simulink model "FixedWing_Dynamic_Model_SIL_simulink"  (R2023a)
settings: Solver=ode4  StartTime=0.0  StopTime=timestop  FixedStep=0.004  RelTol=1e-3
model workspace (MAT data in the model file):
  sample_time = 0.004
values from neighbouring files (symbols this model uses):
  env = struct    [InitEnvironment.m]    (also in resultados_autotuning_H200.mat = )
  F_lat = 1    [autotuning.m]    (also in resultados_autotuning_H200.mat)
  F_lon = 1    [autotuning.m]    (also in resultados_autotuning_H200.mat)
  frecuency = 0.012    [PX4_var_controllers.m]    (also in resultados_autotuning_H200.mat)
  g = 9.81    [PX4_var_controllers.m]    (also in resultados_autotuning_H200.mat)
  LC =     [resultados_autotuning_H200.mat]
  mission = [wp]    [PX4_var_controllers.m]    (also in resultados_autotuning_H200.mat = )
  nav = 0    [autotuning.m]    (also in resultados_autotuning_H200.mat)
  nwap = 9    [PX4_var_controllers.m]    (also in resultados_autotuning_H200.mat)
  pitch_D = p(8)    [Error_Medio_Cuadratico_tot.m]    (also in autotuning.m = gaDat3.xmin(8); resultados_autotuning_H200.mat = 0.0563748318956)
  pitch_ff = p(10)    [Error_Medio_Cuadratico_tot.m]    (also in autotuning.m = gaDat3.xmin(10); resultados_autotuning_H200.mat = 0.191071934851)
  pitch_I = p(7)    [Error_Medio_Cuadratico_tot.m]    (also in autotuning.m = gaDat3.xmin(7); resultados_autotuning_H200.mat = 5.51002123548)
  pitch_P = p(6)    [Error_Medio_Cuadratico_tot.m]    (also in autotuning.m = gaDat3.xmin(6); resultados_autotuning_H200.mat = 0.842081867818)
  poswp = [poswp1;poswp2;poswp3;poswp4;poswp5;poswp6;poswp7;poswp8;poswp9]    [PX4_var_controllers.m]    (also in resultados_autotuning_H200.mat = [0 203.689232032 39.9384744604 259.790159417 479.641844374 3)
  ref_height = 171    [resultados_autotuning_H200.mat]
  ref_lat = 39.4973880749    [resultados_autotuning_H200.mat]
  ref_lon = -0.626812248872    [resultados_autotuning_H200.mat]
  roll_D = p(3)    [Error_Medio_Cuadratico_lat.m]    (also in Error_Medio_Cuadratico_tot.m; autotuning.m = gaDat3.xmin(3); resultados_autotuning_H200.mat = 0.0337053005157)
  roll_ff = p(5)    [Error_Medio_Cuadratico_lat.m]    (also in Error_Medio_Cuadratico_tot.m; autotuning.m = gaDat3.xmin(5); resultados_autotuning_H200.mat = 0.350805641616)
  roll_I = p(2)    [Error_Medio_Cuadratico_lat.m]    (also in Error_Medio_Cuadratico_tot.m; autotuning.m = gaDat3.xmin(2); resultados_autotuning_H200.mat = 5.74910821603)
  roll_P = p(1)    [Error_Medio_Cuadratico_lat.m]    (also in Error_Medio_Cuadratico_tot.m; autotuning.m = gaDat3.xmin(1); resultados_autotuning_H200.mat = 0.613573974385)
  tc_pitch = p(9)    [Error_Medio_Cuadratico_tot.m]    (also in autotuning.m = gaDat3.xmin(9); resultados_autotuning_H200.mat = 0.651709962584)
  tc_roll = p(4)    [Error_Medio_Cuadratico_lat.m]    (also in Error_Medio_Cuadratico_tot.m; autotuning.m = gaDat3.xmin(4); resultados_autotuning_H200.mat = 0.630975334126)
  TEBCL =     [resultados_autotuning_H200.mat]
  TECL =     [resultados_autotuning_H200.mat]
  TECS =     [resultados_autotuning_H200.mat]
  throttle_sp = 0.6    [autotuning.m]    (also in resultados_autotuning_H200.mat)
  uavData = struct    [InitFixedWingParam.m]    (also in resultados_autotuning_H200.mat = )
  V_cruise = [15,15,15,20,25,25,20,15,15]    [PX4_var_controllers.m]    (also in resultados_autotuning_H200.mat = [15 15 15 20 25 25 20 15 15])
  yaw_D = p(8)    [Error_Medio_Cuadratico_lat.m]    (also in Error_Medio_Cuadratico_tot.m = p(13); autotuning.m = gaDat3.xmin(13); resultados_autotuning_H200.mat = 0.366142516918)
  yaw_ff = p(9)    [Error_Medio_Cuadratico_lat.m]    (also in Error_Medio_Cuadratico_tot.m = p(14); autotuning.m = gaDat3.xmin(14); resultados_autotuning_H200.mat = 1.32395168)
  yaw_I = p(7)    [Error_Medio_Cuadratico_lat.m]    (also in Error_Medio_Cuadratico_tot.m = p(12); autotuning.m = gaDat3.xmin(12); resultados_autotuning_H200.mat = 9.97252106698)
  yaw_P = p(6)    [Error_Medio_Cuadratico_lat.m]    (also in Error_Medio_Cuadratico_tot.m = p(11); autotuning.m = gaDat3.xmin(11); resultados_autotuning_H200.mat = 9.79447138521)
undefined symbols (not defined in the file or in its folder): DiscIntNeverNeededParam, Earth, WGS84
libraries: aerolibactuator x5, aerolibasang x4, slpidlib x3, uavalgslib x2, aerolibatmos2 x2, shared6dof x1, aerolibtransform2 x1, simulink_extras x1
(part 3 of 3)

== system FixedWing_Dynamic_Model_SIL_simulink/Dynamics/H200 Fixed-wing UAV Dynamics/Force and Moment Calculation/Motor Model/Engine Model/Thurst Model/N [Hz] model ==
  deltaP : Inport
  " " : Gain  Gain=uavData.engine.propellerModel.RPMModel.pn1
  Saturation : Saturate  UpperLimit=1  LowerLimit=0
  n : Outport
  wires:
  " "/1 -> n/1
  deltaP/1 -> Saturation/1
  Saturation/1 -> " "/1

== system FixedWing_Dynamic_Model_SIL_simulink/Dynamics/H200 Fixed-wing UAV Dynamics/Force and Moment Calculation/Motor Model/Engine Model/Thurst Model/Thrust Force ==
  n : Inport
  CT : Inport  Port=2
  rho : Inport  Port=3
  Constant : Constant  Value=uavData.engine.bladeDiameter
  Constant1 : Constant  Value=4
  Power : Math  Operator=pow
  Product : Product  Inputs=4
  Square : Math  Operator=square
  T : Outport
  wires:
  Constant/1 -> Power/1
  n/1 -> Square/1
  Square/1 -> Product/1
  CT/1 -> Product/2
  rho/1 -> Product/3
  Product/1 -> T/1
  Power/1 -> Product/4
  Constant1/1 -> Power/2

== system FixedWing_Dynamic_Model_SIL_simulink/Dynamics/H200 Fixed-wing UAV Dynamics/Force and Moment Calculation/Aerodynamic Forces and Moments/Compute Body Frame Forces and Moments/Rotate FM to body frame/Rotate Forces/RB2W ==
  aoa beta : Inport
  11 : Fcn  Expr=u[3]*u[4]
  12 : Fcn  Expr=u[2]
  13 : Fcn  Expr=u[1]*u[4]
  21 : Fcn  Expr=-u[3]*u[2]
  22 : Fcn  Expr=u[4]
  23 : Fcn  Expr=-u[1]*u[2]
  31 : Fcn  Expr=-u[1]
  32 : Fcn  Expr=0
  33 : Fcn  Expr=u[3]
  Mux : Mux  Inputs=2
  Mux3 : Mux  Inputs=9
  Reshape 9x1->3x3 : Reshape  OutputDimensionality=Customize  OutputDimensions=[3,3]
  sincos : Trigonometry  Operator=sincos
  Rw2b : Outport  VectorParamsAs1DForOutWhenUnconnected=off
  wires:
  Mux/1 -> 11/1, 21/1, 31/1, 12/1, 22/1, 32/1, 13/1, 23/1, 33/1
  aoa beta/1 -> sincos/1
  sincos/2 -> Mux/2
  sincos/1 -> Mux/1
  33/1 -> Mux3/9
  23/1 -> Mux3/8
  13/1 -> Mux3/7
  32/1 -> Mux3/6
  22/1 -> Mux3/5
  12/1 -> Mux3/4
  31/1 -> Mux3/3
  21/1 -> Mux3/2
  11/1 -> Mux3/1
  Reshape 9x1->3x3/1 -> Rw2b/1
  Mux3/1 -> Reshape 9x1->3x3/1

== system FixedWing_Dynamic_Model_SIL_simulink/Dynamics/H200 Fixed-wing UAV Dynamics/Force and Moment Calculation/Aerodynamic Forces and Moments/Compute Body Frame Forces and Moments/Rotate FM to body frame/Rotate Moments/RB2W ==
  aoa beta : Inport
  11 : Fcn  Expr=u[3]*u[4]
  12 : Fcn  Expr=u[2]
  13 : Fcn  Expr=u[1]*u[4]
  21 : Fcn  Expr=-u[3]*u[2]
  22 : Fcn  Expr=u[4]
  23 : Fcn  Expr=-u[1]*u[2]
  31 : Fcn  Expr=-u[1]
  32 : Fcn  Expr=0
  33 : Fcn  Expr=u[3]
  Mux : Mux  Inputs=2
  Mux3 : Mux  Inputs=9
  Reshape 9x1->3x3 : Reshape  OutputDimensionality=Customize  OutputDimensions=[3,3]
  sincos : Trigonometry  Operator=sincos
  Rw2b : Outport  VectorParamsAs1DForOutWhenUnconnected=off
  wires:
  Mux/1 -> 11/1, 21/1, 31/1, 12/1, 22/1, 32/1, 13/1, 23/1, 33/1
  aoa beta/1 -> sincos/1
  sincos/2 -> Mux/2
  sincos/1 -> Mux/1
  33/1 -> Mux3/9
  23/1 -> Mux3/8
  13/1 -> Mux3/7
  32/1 -> Mux3/6
  22/1 -> Mux3/5
  12/1 -> Mux3/4
  31/1 -> Mux3/3
  21/1 -> Mux3/2
  11/1 -> Mux3/1
  Reshape 9x1->3x3/1 -> Rw2b/1
  Mux3/1 -> Reshape 9x1->3x3/1

== system FixedWing_Dynamic_Model_SIL_simulink/Dynamics/H200 Fixed-wing UAV Dynamics/Force and Moment Calculation/Aerodynamic Forces and Moments/Compute Body Frame Forces and Moments/Wind frame F& M/Lateral Channel/CY ==
  beta : Inport
  p,q,r : Inport  Port=2
  Airspeed : Inport  Port=3
  deltaR : Inport  Port=4
  deltaA : Inport  Port=5
  CYDr : Constant  Value=uavData.aero.CYdeltaR
      settings: AttributesFormatString=%<Value>
  CYDr1 : Constant  Value=uavData.aero.CYdeltaA
      settings: AttributesFormatString=%<Value>
  CYb : Constant  Value=uavData.aero.CYbeta
      settings: AttributesFormatString=%<Value>
  Product : Product  SaturateOnIntegerOverflow=on  OutDataTypeStr=Inherit: Same as first input
  Product1 : Product  SaturateOnIntegerOverflow=on  OutDataTypeStr=Inherit: Same as first input
  Product2 : Product  SaturateOnIntegerOverflow=on  OutDataTypeStr=Inherit: Same as first input
  Sum2 : Sum  Inputs=+++++  SaturateOnIntegerOverflow=on
  roll / yaw rate factors : Subsystem
  CY : Outport  VectorParamsAs1DForOutWhenUnconnected=off
  wires:
  deltaR/1 -> Product1/2
  CYDr/1 -> Product1/1
  Product/1 -> Sum2/1
  Sum2/1 -> CY/1
  beta/1 -> Product/2
  CYb/1 -> Product/1
  CYDr1/1 -> Product2/1
  deltaA/1 -> Product2/2
  Product2/1 -> Sum2/5
  Product1/1 -> Sum2/4
  roll / yaw rate factors/1(CYp) -> Sum2/2
  roll / yaw rate factors/2(CYr) -> Sum2/3
  p,q,r/1 -> roll / yaw rate factors/1(p,q,r)
  Airspeed/1 -> roll / yaw rate factors/2(Airspeed)

== system FixedWing_Dynamic_Model_SIL_simulink/Dynamics/H200 Fixed-wing UAV Dynamics/Force and Moment Calculation/Aerodynamic Forces and Moments/Compute Body Frame Forces and Moments/Wind frame F& M/Lateral Channel/Cl ==
  beta : Inport
  p,q,r : Inport  Port=2
  Airspeed : Inport  Port=3
  deltaR : Inport  Port=4
  deltaA : Inport  Port=5
  CYDr : Constant  Value=uavData.aero.CldeltaR
      settings: AttributesFormatString=%<Value>
  CYDr1 : Constant  Value=uavData.aero.CldeltaA
      settings: AttributesFormatString=%<Value>
  Clb : Constant  Value=uavData.aero.Clbeta
      settings: AttributesFormatString=%<Value>
  Product2 : Product  SaturateOnIntegerOverflow=on  OutDataTypeStr=Inherit: Same as first input
  Product3 : Product  SaturateOnIntegerOverflow=on  OutDataTypeStr=Inherit: Same as first input
  Product4 : Product  SaturateOnIntegerOverflow=on  OutDataTypeStr=Inherit: Same as first input
  Sum : Sum  Inputs=+++++  SaturateOnIntegerOverflow=on
  roll factors : Subsystem
  Cl : Outport  VectorParamsAs1DForOutWhenUnconnected=off
  wires:
  Airspeed/1 -> roll factors/2(Airspeed)
  p,q,r/1 -> roll factors/1(p,q,r)
  Product4/1 -> Sum/1  "Clb"
  Sum/1 -> Cl/1
  beta/1 -> Product4/2
  Clb/1 -> Product4/1
  CYDr1/1 -> Product3/1
  deltaR/1 -> Product2/2
  deltaA/1 -> Product3/2
  Product2/1 -> Sum/4
  CYDr/1 -> Product2/1
  Product3/1 -> Sum/5
  roll factors/1(Clp) -> Sum/2
  roll factors/2(Clr) -> Sum/3

== system FixedWing_Dynamic_Model_SIL_simulink/Dynamics/H200 Fixed-wing UAV Dynamics/Force and Moment Calculation/Aerodynamic Forces and Moments/Compute Body Frame Forces and Moments/Wind frame F& M/Lateral Channel/Cn ==
  beta : Inport
  p,q,r : Inport  Port=2
  Airspeed : Inport  Port=3
  deltaR : Inport  Port=4
  deltaA : Inport  Port=5
  CnDa : Constant  Value=uavData.aero.CndeltaA
      settings: AttributesFormatString=%<Value>
  CnDr : Constant  Value=uavData.aero.CndeltaR
      settings: AttributesFormatString=%<Value>
  Cnb : Constant  Value=uavData.aero.Cnbeta
      settings: AttributesFormatString=%<Value>
  Product2 : Product  SaturateOnIntegerOverflow=on  OutDataTypeStr=Inherit: Same as first input
  Product3 : Product  SaturateOnIntegerOverflow=on  OutDataTypeStr=Inherit: Same as first input
  Product4 : Product  SaturateOnIntegerOverflow=on  OutDataTypeStr=Inherit: Same as first input
  Sum : Sum  Inputs=+++++  SaturateOnIntegerOverflow=on
  roll / yaw rate factors : Subsystem
  Cn : Outport  VectorParamsAs1DForOutWhenUnconnected=off
  wires:
  Airspeed/1 -> roll / yaw rate factors/2(Airspeed)
  p,q,r/1 -> roll / yaw rate factors/1(p,q,r)
  Cnb/1 -> Product4/1
  beta/1 -> Product4/2
  Sum/1 -> Cn/1
  Product4/1 -> Sum/1
  roll / yaw rate factors/1(Cnp) -> Sum/2
  roll / yaw rate factors/2(Cnr) -> Sum/3
  deltaR/1 -> Product2/2
  CnDr/1 -> Product2/1
  CnDa/1 -> Product3/1
  deltaA/1 -> Product3/2
  Product2/1 -> Sum/4
  Product3/1 -> Sum/5

== system FixedWing_Dynamic_Model_SIL_simulink/Dynamics/H200 Fixed-wing UAV Dynamics/Force and Moment Calculation/Aerodynamic Forces and Moments/Compute Body Frame Forces and Moments/Wind frame F& M/Longitudinal Channel/CD ==
  CL : Inport
  Apolar : Constant  Value=uavData.aero.A1
      settings: AttributesFormatString=%<Value>
  Apolar (A2) : Constant  Value=uavData.aero.Apolar
      settings: AttributesFormatString=%<Value>
  CD0 : Constant  Value=uavData.aero.CD0
      settings: AttributesFormatString=%<Value>
  Math Function : Math  Operator=square  SignedPower=on
  Product : Product  SaturateOnIntegerOverflow=on  OutDataTypeStr=Inherit: Same as first input
  Product1 : Product  SaturateOnIntegerOverflow=on  OutDataTypeStr=Inherit: Same as first input
  Sum1 : Sum  Inputs=+++  SaturateOnIntegerOverflow=on
  CD : Outport  VectorParamsAs1DForOutWhenUnconnected=off
  wires:
  Sum1/1 -> CD/1
  Apolar (A2)/1 -> Product/1
  Math Function/1 -> Product/2
  Product1/1 -> Sum1/3
  Product/1 -> Sum1/2
  CL/1 -> Math Function/1, Product1/1
  CD0/1 -> Sum1/1
  Apolar/1 -> Product1/2

== system FixedWing_Dynamic_Model_SIL_simulink/Dynamics/H200 Fixed-wing UAV Dynamics/Force and Moment Calculation/Aerodynamic Forces and Moments/Compute Body Frame Forces and Moments/Wind frame F& M/Longitudinal Channel/CL ==
  alpha : Inport
  alpha_dot : Inport  Port=2
  p,q,r : Inport  Port=3
  Airspeed : Inport  Port=4
  deltaE : Inport  Port=5
  deltaF : Inport  Port=6
  AoA rate / pitch rate factors : Subsystem
  CL0 : Constant  Value=uavData.aero.CL0
      settings: AttributesFormatString=%<Value>
  CLDe : Constant  Value=uavData.aero.CLdeltaE
      settings: AttributesFormatString=%<Value>
  CLa : Constant  Value=uavData.aero.CLalpha
      settings: AttributesFormatString=%<Value>
  CmDe1 : Constant  Value=uavData.aero.CLdeltaF
      settings: AttributesFormatString=%<Value>
  Product1 : Product  SaturateOnIntegerOverflow=on  OutDataTypeStr=Inherit: Same as first input
  Product3 : Product  SaturateOnIntegerOverflow=on  OutDataTypeStr=Inherit: Same as first input
  Product4 : Product  SaturateOnIntegerOverflow=on  OutDataTypeStr=Inherit: Same as first input
  Sum : Sum  Inputs=++++++  SaturateOnIntegerOverflow=on
  CL : Outport  VectorParamsAs1DForOutWhenUnconnected=off
  wires:
  CL0/1 -> Sum/1  "CL0"
  deltaF/1 -> Product3/2
  Sum/1 -> CL/1
  deltaE/1 -> Product1/2
  CLDe/1 -> Product1/1
  alpha/1 -> Product4/2
  CLa/1 -> Product4/1
  Product4/1 -> Sum/2  "CLalpha"
  alpha_dot/1 -> AoA rate / pitch rate factors/1(alpha_dot)
  Airspeed/1 -> AoA rate / pitch rate factors/3(Airspeed)
  p,q,r/1 -> AoA rate / pitch rate factors/2(p,q,r)
  AoA rate / pitch rate factors/1(CLalpha_dot) -> Sum/3  "CLapha_dot"
  AoA rate / pitch rate factors/2(CLq) -> Sum/4  "CLq"
  Product1/1 -> Sum/5  "CLdeltaE"
  CmDe1/1 -> Product3/1
  Product3/1 -> Sum/6  "CLdeltaF"

== system FixedWing_Dynamic_Model_SIL_simulink/Dynamics/H200 Fixed-wing UAV Dynamics/Force and Moment Calculation/Aerodynamic Forces and Moments/Compute Body Frame Forces and Moments/Wind frame F& M/Longitudinal Channel/Cm ==
  alpha : Inport
  alpha_dot : Inport  Port=2
  p,q,r : Inport  Port=3
  Airpseed : Inport  Port=4
  deltaE : Inport  Port=5
  deltaF : Inport  Port=6
  AoA rate / pitch rate factors : Subsystem
  Cm0 : Constant  Value=uavData.aero.Cm0
      settings: AttributesFormatString=%<Value>
  CmDe : Constant  Value=uavData.aero.CmdeltaE
      settings: AttributesFormatString=%<Value>
  CmDf : Constant  Value=uavData.aero.CmdeltaF
      settings: AttributesFormatString=%<Value>
  Cma : Constant  Value=uavData.aero.Cmalpha
      settings: AttributesFormatString=%<Value>
  Product1 : Product  Inputs=***/  SaturateOnIntegerOverflow=on  OutDataTypeStr=Inherit: Same as first input
  Product2 : Product  SaturateOnIntegerOverflow=on  OutDataTypeStr=Inherit: Same as first input
  Product4 : Product  SaturateOnIntegerOverflow=on  OutDataTypeStr=Inherit: Same as first input
  Sum : Sum  Inputs=++++++  SaturateOnIntegerOverflow=on
  chord : Constant  Value=uavData.geometry.cw
      settings: AttributesFormatString=%<Value>
  elarm : Constant  Value=uavData.geometry.LElev
      settings: AttributesFormatString=%<Value>
  Cm : Outport  VectorParamsAs1DForOutWhenUnconnected=off
  wires:
  chord/1 -> Product1/4
  elarm/1 -> Product1/3
  Product4/1 -> Sum/2  "cma"
  Sum/1 -> Cm/1  "total"
  deltaE/1 -> Product1/2
  CmDe/1 -> Product1/1
  alpha/1 -> Product4/2
  Cma/1 -> Product4/1
  deltaF/1 -> Product2/2
  CmDf/1 -> Product2/1
  Cm0/1 -> Sum/1  "cm0"
  alpha_dot/1 -> AoA rate / pitch rate factors/1(alpha_dot)
  p,q,r/1 -> AoA rate / pitch rate factors/2(p,q,r)
  Airpseed/1 -> AoA rate / pitch rate factors/3(Airspeed)
  AoA rate / pitch rate factors/1(Cmalpha_dot) -> Sum/3  "Cmalpha_dot"
  AoA rate / pitch rate factors/2(Cmq) -> Sum/4  "Cmq"
  Product1/1 -> Sum/5  "cmde"
  Product2/1 -> Sum/6  "cmdf"

== system FixedWing_Dynamic_Model_SIL_simulink/Dynamics/H200 Fixed-wing UAV Dynamics/Force and Moment Calculation/Aerodynamic Forces and Moments/Compute Body Frame Forces and Moments/Wind frame F& M/Lateral Channel/CY/roll // yaw rate factors ==
  p,q,r : Inport
  Airspeed : Inport  Port=2
  Constant : Constant  Value=uavData.aero.CYp
      settings: AttributesFormatString=%<Value>
  Constant1 : Constant  Value=uavData.aero.CYr
      settings: AttributesFormatString=%<Value>
  Get p : Selector  IndexMode=Zero-based  InputPortWidth=3  IndexOptions=Index vector (dialog)  Indices=0  OutputSizes=[(-2)]
  Get r : Selector  IndexMode=Zero-based  InputPortWidth=3  IndexOptions=Index vector (dialog)  Indices=2  OutputSizes=[(-2)]
  Product : Product  SaturateOnIntegerOverflow=on  OutDataTypeStr=Inherit: Same as first input
  Product1 : Product  SaturateOnIntegerOverflow=on  OutDataTypeStr=Inherit: Same as first input
  roll rate fact : Subsystem
  yaw rate fact : Subsystem
  CYp : Outport  VectorParamsAs1DForOutWhenUnconnected=off
  CYr : Outport  Port=2  VectorParamsAs1DForOutWhenUnconnected=off
  wires:
  Airspeed/1 -> roll rate fact/2(Airspeed), yaw rate fact/2(Airspeed)
  Get r/1 -> yaw rate fact/1(r)
  p,q,r/1 -> Get p/1, Get r/1
  Get p/1 -> roll rate fact/1(p)
  roll rate fact/1(Roll Rate Fac) -> Product/2
  Constant/1 -> Product/1
  yaw rate fact/1(Yaw Rate Fac) -> Product1/2
  Constant1/1 -> Product1/1
  Product1/1 -> CYr/1
  Product/1 -> CYp/1

== system FixedWing_Dynamic_Model_SIL_simulink/Dynamics/H200 Fixed-wing UAV Dynamics/Force and Moment Calculation/Aerodynamic Forces and Moments/Compute Body Frame Forces and Moments/Wind frame F& M/Lateral Channel/Cl/roll factors ==
  p,q,r : Inport
  Airspeed : Inport  Port=2
  Constant : Constant  Value=uavData.aero.Clp
      settings: AttributesFormatString=%<Value>
  Constant1 : Constant  Value=uavData.aero.Clr
      settings: AttributesFormatString=%<Value>
  Get p : Selector  IndexMode=Zero-based  InputPortWidth=3  IndexOptions=Index vector (dialog)  Indices=0  OutputSizes=[(-2)]
  Get r : Selector  IndexMode=Zero-based  InputPortWidth=3  IndexOptions=Index vector (dialog)  Indices=2  OutputSizes=[(-2)]
  Product : Product  SaturateOnIntegerOverflow=on  OutDataTypeStr=Inherit: Same as first input
  Product1 : Product  SaturateOnIntegerOverflow=on  OutDataTypeStr=Inherit: Same as first input
  roll rate fact : Subsystem
  yaw rate fact : Subsystem
  Clp : Outport  VectorParamsAs1DForOutWhenUnconnected=off
  Clr : Outport  Port=2  VectorParamsAs1DForOutWhenUnconnected=off
  wires:
  Get r/1 -> yaw rate fact/1(r)
  p,q,r/1 -> Get p/1, Get r/1
  Get p/1 -> roll rate fact/1(p)
  Airspeed/1 -> yaw rate fact/2(Airspeed), roll rate fact/2(Airspeed)
  yaw rate fact/1(Yaw Rate Fac) -> Product1/2
  Constant1/1 -> Product1/1
  roll rate fact/1(Roll Rate Fac) -> Product/2
  Constant/1 -> Product/1
  Product1/1 -> Clr/1
  Product/1 -> Clp/1

== system FixedWing_Dynamic_Model_SIL_simulink/Dynamics/H200 Fixed-wing UAV Dynamics/Force and Moment Calculation/Aerodynamic Forces and Moments/Compute Body Frame Forces and Moments/Wind frame F& M/Lateral Channel/Cn/roll // yaw rate factors ==
  p,q,r : Inport
  Airspeed : Inport  Port=2
  Constant : Constant  Value=uavData.aero.Cnp
      settings: AttributesFormatString=%<Value>
  Constant1 : Constant  Value=uavData.aero.Cnr
      settings: AttributesFormatString=%<Value>
  Get p : Selector  IndexMode=Zero-based  InputPortWidth=3  IndexOptions=Index vector (dialog)  Indices=0  OutputSizes=[(-2)]
  Get r : Selector  IndexMode=Zero-based  InputPortWidth=3  IndexOptions=Index vector (dialog)  Indices=2  OutputSizes=[(-2)]
  Product : Product  SaturateOnIntegerOverflow=on  OutDataTypeStr=Inherit: Same as first input
  Product1 : Product  SaturateOnIntegerOverflow=on  OutDataTypeStr=Inherit: Same as first input
  roll rate fact : Subsystem
  yaw rate fact : Subsystem
  Cnp : Outport  VectorParamsAs1DForOutWhenUnconnected=off
  Cnr : Outport  Port=2  VectorParamsAs1DForOutWhenUnconnected=off
  wires:
  Airspeed/1 -> roll rate fact/2(Airspeed), yaw rate fact/2(Airspeed)
  Get r/1 -> yaw rate fact/1(r)
  p,q,r/1 -> Get p/1, Get r/1
  Get p/1 -> roll rate fact/1(p)
  roll rate fact/1(Roll Rate Fac) -> Product/2
  Constant/1 -> Product/1
  yaw rate fact/1(Yaw Rate Fac) -> Product1/2
  Constant1/1 -> Product1/1
  Product1/1 -> Cnr/1
  Product/1 -> Cnp/1

== system FixedWing_Dynamic_Model_SIL_simulink/Dynamics/H200 Fixed-wing UAV Dynamics/Force and Moment Calculation/Aerodynamic Forces and Moments/Compute Body Frame Forces and Moments/Wind frame F& M/Longitudinal Channel/CL/AoA rate // pitch rate factors ==
  alpha_dot : Inport
  p,q,r : Inport  Port=2
  Airspeed : Inport  Port=3
  AoA rate fact : Subsystem
  Constant : Constant  Value=uavData.aero.CLalpha_dot
      settings: AttributesFormatString=%<Value>
  Constant1 : Constant  Value=uavData.aero.CLq
      settings: AttributesFormatString=%<Value>
  Get r : Selector  IndexMode=Zero-based  InputPortWidth=3  IndexOptions=Index vector (dialog)  Indices=1  OutputSizes=[(-2)]
  Product : Product  SaturateOnIntegerOverflow=on  OutDataTypeStr=Inherit: Same as first input
  Product1 : Product  SaturateOnIntegerOverflow=on  OutDataTypeStr=Inherit: Same as first input
  roll rate fact : Subsystem
  CLalpha_dot : Outport  VectorParamsAs1DForOutWhenUnconnected=off
  CLq : Outport  Port=2  VectorParamsAs1DForOutWhenUnconnected=off
  wires:
  Airspeed/1 -> roll rate fact/2(Airspeed), AoA rate fact/2(Airspeed)
  Get r/1 -> roll rate fact/1(q)
  p,q,r/1 -> Get r/1
  AoA rate fact/1(AoA Rate Fac) -> Product/2
  Constant/1 -> Product/1
  roll rate fact/1(Roll Rate Fac) -> Product1/2
  Constant1/1 -> Product1/1
  Product1/1 -> CLq/1
  Product/1 -> CLalpha_dot/1
  alpha_dot/1 -> AoA rate fact/1(alpha_dot)

== system FixedWing_Dynamic_Model_SIL_simulink/Dynamics/H200 Fixed-wing UAV Dynamics/Force and Moment Calculation/Aerodynamic Forces and Moments/Compute Body Frame Forces and Moments/Wind frame F& M/Longitudinal Channel/Cm/AoA rate // pitch rate factors ==
  alpha_dot : Inport
  p,q,r : Inport  Port=2
  Airspeed : Inport  Port=3
  AoA rate fact : Subsystem
  Constant : Constant  Value=uavData.aero.Cmalpha_dot
      settings: AttributesFormatString=%<Value>
  Constant1 : Constant  Value=uavData.aero.Cmq
      settings: AttributesFormatString=%<Value>
  Get r : Selector  IndexMode=Zero-based  InputPortWidth=3  IndexOptions=Index vector (dialog)  Indices=1  OutputSizes=[(-2)]
  Product : Product  SaturateOnIntegerOverflow=on  OutDataTypeStr=Inherit: Same as first input
  Product1 : Product  SaturateOnIntegerOverflow=on  OutDataTypeStr=Inherit: Same as first input
  pitch rate fact : Subsystem
  Cmalpha_dot : Outport  VectorParamsAs1DForOutWhenUnconnected=off
  Cmq : Outport  Port=2  VectorParamsAs1DForOutWhenUnconnected=off
  wires:
  Airspeed/1 -> pitch rate fact/2(Airspeed), AoA rate fact/2(Airspeed)
  Get r/1 -> pitch rate fact/1(q)
  p,q,r/1 -> Get r/1
  AoA rate fact/1(AoA Rate Fac) -> Product/2
  Constant/1 -> Product/1
  pitch rate fact/1(Pitch Rate Fac) -> Product1/2
  Constant1/1 -> Product1/1
  Product1/1 -> Cmq/1
  Product/1 -> Cmalpha_dot/1
  alpha_dot/1 -> AoA rate fact/1(alpha_dot)

== system FixedWing_Dynamic_Model_SIL_simulink/Dynamics/H200 Fixed-wing UAV Dynamics/Force and Moment Calculation/Aerodynamic Forces and Moments/Compute Body Frame Forces and Moments/Wind frame F& M/Lateral Channel/CY/roll // yaw rate factors/roll rate fact ==
  p : Inport
  Airspeed : Inport  Port=2
  Cmq1 : Constant  Value=.5
      settings: AttributesFormatString=%<Value>
  Cmq2 : Constant  Value=uavData.geometry.bw
      settings: AttributesFormatString=%<Value>
  Product : Product  Inputs=***/  SaturateOnIntegerOverflow=on  OutDataTypeStr=Inherit: Same as first input
  Saturation : Saturate  UpperLimit=inf  LowerLimit=0.1
      settings: AttributesFormatString="[%<LowerLimit>  %<UpperLimit>]"
  Roll Rate Fac : Outport  VectorParamsAs1DForOutWhenUnconnected=off
  wires:
  Saturation/1 -> Product/4
  Airspeed/1 -> Saturation/1
  Cmq2/1 -> Product/3
  Cmq1/1 -> Product/2
  p/1 -> Product/1
  Product/1 -> Roll Rate Fac/1

== system FixedWing_Dynamic_Model_SIL_simulink/Dynamics/H200 Fixed-wing UAV Dynamics/Force and Moment Calculation/Aerodynamic Forces and Moments/Compute Body Frame Forces and Moments/Wind frame F& M/Lateral Channel/CY/roll // yaw rate factors/yaw rate fact ==
  r : Inport
  Airspeed : Inport  Port=2
  Cmq3 : Constant  Value=.5
      settings: AttributesFormatString=%<Value>
  Cmq4 : Constant  Value=uavData.geometry.bw
      settings: AttributesFormatString=%<Value>
  Product1 : Product  Inputs=***/  SaturateOnIntegerOverflow=on  OutDataTypeStr=Inherit: Same as first input
  Saturation : Saturate  UpperLimit=inf  LowerLimit=0.1
      settings: AttributesFormatString="[%<LowerLimit>  %<UpperLimit>]"
  Yaw Rate Fac : Outport  VectorParamsAs1DForOutWhenUnconnected=off
  wires:
  Product1/1 -> Yaw Rate Fac/1
  r/1 -> Product1/1
  Cmq3/1 -> Product1/2
  Cmq4/1 -> Product1/3
  Airspeed/1 -> Saturation/1
  Saturation/1 -> Product1/4

== system FixedWing_Dynamic_Model_SIL_simulink/Dynamics/H200 Fixed-wing UAV Dynamics/Force and Moment Calculation/Aerodynamic Forces and Moments/Compute Body Frame Forces and Moments/Wind frame F& M/Lateral Channel/Cl/roll factors/roll rate fact ==
  p : Inport
  Airspeed : Inport  Port=2
  Cmq1 : Constant  Value=.5
      settings: AttributesFormatString=%<Value>
  Cmq2 : Constant  Value=uavData.geometry.bw
      settings: AttributesFormatString=%<Value>
  Product : Product  Inputs=***/  SaturateOnIntegerOverflow=on  OutDataTypeStr=Inherit: Same as first input
  Saturation : Saturate  UpperLimit=inf  LowerLimit=0.1
      settings: AttributesFormatString="[%<LowerLimit>  %<UpperLimit>]"
  Roll Rate Fac : Outport  VectorParamsAs1DForOutWhenUnconnected=off
  wires:
  Saturation/1 -> Product/4
  Airspeed/1 -> Saturation/1
  Cmq2/1 -> Product/3
  Cmq1/1 -> Product/2
  p/1 -> Product/1
  Product/1 -> Roll Rate Fac/1

== system FixedWing_Dynamic_Model_SIL_simulink/Dynamics/H200 Fixed-wing UAV Dynamics/Force and Moment Calculation/Aerodynamic Forces and Moments/Compute Body Frame Forces and Moments/Wind frame F& M/Lateral Channel/Cl/roll factors/yaw rate fact ==
  r : Inport
  Airspeed : Inport  Port=2
  Cmq3 : Constant  Value=.5
      settings: AttributesFormatString=%<Value>
  Cmq4 : Constant  Value=uavData.geometry.bw
      settings: AttributesFormatString=%<Value>
  Product1 : Product  Inputs=***/  SaturateOnIntegerOverflow=on  OutDataTypeStr=Inherit: Same as first input
  Saturation : Saturate  UpperLimit=inf  LowerLimit=0.1
      settings: AttributesFormatString="[%<LowerLimit>  %<UpperLimit>]"
  Yaw Rate Fac : Outport  VectorParamsAs1DForOutWhenUnconnected=off
  wires:
  Product1/1 -> Yaw Rate Fac/1
  r/1 -> Product1/1
  Cmq3/1 -> Product1/2
  Cmq4/1 -> Product1/3
  Airspeed/1 -> Saturation/1
  Saturation/1 -> Product1/4

== system FixedWing_Dynamic_Model_SIL_simulink/Dynamics/H200 Fixed-wing UAV Dynamics/Force and Moment Calculation/Aerodynamic Forces and Moments/Compute Body Frame Forces and Moments/Wind frame F& M/Lateral Channel/Cn/roll // yaw rate factors/roll rate fact ==
  p : Inport
  Airspeed : Inport  Port=2
  Cmq1 : Constant  Value=.5
      settings: AttributesFormatString=%<Value>
  Cmq2 : Constant  Value=uavData.geometry.bw
      settings: AttributesFormatString=%<Value>
  Product : Product  Inputs=***/  SaturateOnIntegerOverflow=on  OutDataTypeStr=Inherit: Same as first input
  Saturation : Saturate  UpperLimit=inf  LowerLimit=0.1
      settings: AttributesFormatString="[%<LowerLimit>  %<UpperLimit>]"
  Roll Rate Fac : Outport  VectorParamsAs1DForOutWhenUnconnected=off
  wires:
  Saturation/1 -> Product/4
  Airspeed/1 -> Saturation/1
  Cmq2/1 -> Product/3
  Cmq1/1 -> Product/2
  p/1 -> Product/1
  Product/1 -> Roll Rate Fac/1

== system FixedWing_Dynamic_Model_SIL_simulink/Dynamics/H200 Fixed-wing UAV Dynamics/Force and Moment Calculation/Aerodynamic Forces and Moments/Compute Body Frame Forces and Moments/Wind frame F& M/Lateral Channel/Cn/roll // yaw rate factors/yaw rate fact ==
  r : Inport
  Airspeed : Inport  Port=2
  Cmq3 : Constant  Value=.5
      settings: AttributesFormatString=%<Value>
  Cmq4 : Constant  Value=uavData.geometry.bw
      settings: AttributesFormatString=%<Value>
  Product1 : Product  Inputs=***/  SaturateOnIntegerOverflow=on  OutDataTypeStr=Inherit: Same as first input
  Saturation : Saturate  UpperLimit=inf  LowerLimit=0.1
      settings: AttributesFormatString="[%<LowerLimit>  %<UpperLimit>]"
  Yaw Rate Fac : Outport  VectorParamsAs1DForOutWhenUnconnected=off
  wires:
  Product1/1 -> Yaw Rate Fac/1
  r/1 -> Product1/1
  Cmq3/1 -> Product1/2
  Cmq4/1 -> Product1/3
  Airspeed/1 -> Saturation/1
  Saturation/1 -> Product1/4

== system FixedWing_Dynamic_Model_SIL_simulink/Dynamics/H200 Fixed-wing UAV Dynamics/Force and Moment Calculation/Aerodynamic Forces and Moments/Compute Body Frame Forces and Moments/Wind frame F& M/Longitudinal Channel/CL/AoA rate // pitch rate factors/AoA rate fact ==
  alpha_dot : Inport
  Airspeed : Inport  Port=2
  Cmq1 : Constant  Value=.5
      settings: AttributesFormatString=%<Value>
  Cmq2 : Constant  Value=uavData.geometry.cw
      settings: AttributesFormatString=%<Value>
  Product : Product  Inputs=***/  SaturateOnIntegerOverflow=on  OutDataTypeStr=Inherit: Same as first input
  Saturation : Saturate  UpperLimit=inf  LowerLimit=0.1
      settings: AttributesFormatString="[%<LowerLimit>  %<UpperLimit>]"
  AoA Rate Fac : Outport  VectorParamsAs1DForOutWhenUnconnected=off
  wires:
  Saturation/1 -> Product/4
  Airspeed/1 -> Saturation/1
  Cmq2/1 -> Product/3
  Cmq1/1 -> Product/2
  alpha_dot/1 -> Product/1
  Product/1 -> AoA Rate Fac/1

== system FixedWing_Dynamic_Model_SIL_simulink/Dynamics/H200 Fixed-wing UAV Dynamics/Force and Moment Calculation/Aerodynamic Forces and Moments/Compute Body Frame Forces and Moments/Wind frame F& M/Longitudinal Channel/CL/AoA rate // pitch rate factors/roll rate fact ==
  q : Inport
  Airspeed : Inport  Port=2
  Cmq3 : Constant  Value=.5
      settings: AttributesFormatString=%<Value>
  Cmq4 : Constant  Value=uavData.geometry.cw
      settings: AttributesFormatString=%<Value>
  Product1 : Product  Inputs=***/  SaturateOnIntegerOverflow=on  OutDataTypeStr=Inherit: Same as first input
  Saturation : Saturate  UpperLimit=inf  LowerLimit=0.1
      settings: AttributesFormatString="[%<LowerLimit>  %<UpperLimit>]"
  Roll Rate Fac : Outport  VectorParamsAs1DForOutWhenUnconnected=off
  wires:
  Product1/1 -> Roll Rate Fac/1
  q/1 -> Product1/1
  Cmq3/1 -> Product1/2
  Cmq4/1 -> Product1/3
  Airspeed/1 -> Saturation/1
  Saturation/1 -> Product1/4

== system FixedWing_Dynamic_Model_SIL_simulink/Dynamics/H200 Fixed-wing UAV Dynamics/Force and Moment Calculation/Aerodynamic Forces and Moments/Compute Body Frame Forces and Moments/Wind frame F& M/Longitudinal Channel/Cm/AoA rate // pitch rate factors/AoA rate fact ==
  alpha_dot : Inport
  Airspeed : Inport  Port=2
  Cmq1 : Constant  Value=.5
      settings: AttributesFormatString=%<Value>
  Cmq2 : Constant  Value=uavData.geometry.cw
      settings: AttributesFormatString=%<Value>
  Product : Product  Inputs=***/  SaturateOnIntegerOverflow=on  OutDataTypeStr=Inherit: Same as first input
  Saturation : Saturate  UpperLimit=inf  LowerLimit=0.1
      settings: AttributesFormatString="[%<LowerLimit>  %<UpperLimit>]"
  AoA Rate Fac : Outport  VectorParamsAs1DForOutWhenUnconnected=off
  wires:
  Saturation/1 -> Product/4
  Airspeed/1 -> Saturation/1
  Cmq2/1 -> Product/3
  Cmq1/1 -> Product/2
  alpha_dot/1 -> Product/1
  Product/1 -> AoA Rate Fac/1

== system FixedWing_Dynamic_Model_SIL_simulink/Dynamics/H200 Fixed-wing UAV Dynamics/Force and Moment Calculation/Aerodynamic Forces and Moments/Compute Body Frame Forces and Moments/Wind frame F& M/Longitudinal Channel/Cm/AoA rate // pitch rate factors/pitch rate fact ==
  q : Inport
  Airspeed : Inport  Port=2
  Cmq3 : Constant  Value=.5
      settings: AttributesFormatString=%<Value>
  Cmq4 : Constant  Value=uavData.geometry.cw
      settings: AttributesFormatString=%<Value>
  Product1 : Product  Inputs=***/  SaturateOnIntegerOverflow=on  OutDataTypeStr=Inherit: Same as first input
  Saturation : Saturate  UpperLimit=inf  LowerLimit=0.1
      settings: AttributesFormatString="[%<LowerLimit>  %<UpperLimit>]"
  Pitch Rate Fac : Outport  VectorParamsAs1DForOutWhenUnconnected=off
  wires:
  Product1/1 -> Pitch Rate Fac/1
  q/1 -> Product1/1
  Cmq3/1 -> Product1/2
  Cmq4/1 -> Product1/3
  Airspeed/1 -> Saturation/1
  Saturation/1 -> Product1/4

== matlab function FixedWing_Dynamic_Model_SIL_simulink/Controllers/Total Energy control system/Total energy balance control loop/MATLAB Function1 ==
  data: SEB_rate_correction input; pitch_setpoint_1 output; V_TAS input
function pitch_setpoint_1  = seb_to_pitch(SEB_rate_correction,V_TAS)

g = 9.81;
airspeed_for_seb_rate = 15;

if V_TAS > 10^-6

airspeed_for_seb_rate = V_TAS;
end 

climb_angle_to_SEB_rate = airspeed_for_seb_rate*g;

pitch_setpoint_1 = SEB_rate_correction/climb_angle_to_SEB_rate;

== matlab function FixedWing_Dynamic_Model_SIL_simulink/Controllers/L1 Controller/MATLAB Function1 ==
  data: eta input; eta output
function eta = fcn(eta)
eta = mod(eta,2*pi);
if eta>pi
    eta = eta-2*pi;
end

== matlab function FixedWing_Dynamic_Model_SIL_simulink/Controllers/Attitude Controller/MATLAB Function2 ==
  data: roll_setpoint input; roll_body_rate_setpoint_raw output; roll input; euler_yaw_rate_setpoint input; tc input; pitch input
function roll_body_rate_setpoint_raw = roll_crtl(roll_setpoint,roll,euler_yaw_rate_setpoint,tc,pitch)
roll_error = roll_setpoint-roll;
euler_rate_setpoint = roll_error /tc;
roll_body_rate_setpoint_raw = euler_rate_setpoint - sin(pitch)*euler_yaw_rate_setpoint;

== matlab function FixedWing_Dynamic_Model_SIL_simulink/Controllers/Attitude Controller/MATLAB Function3 ==
  data: pitch_body_rate_setpoint_raw output; pitch input; euler_yaw_rate_setpoint input; roll input; euler_rate_setpoint_pitch input
function pitch_body_rate_setpoint_raw  = pitch_crtl(pitch,euler_yaw_rate_setpoint,roll,euler_rate_setpoint_pitch)

pitch_body_rate_setpoint_raw = cos(roll)*euler_rate_setpoint_pitch+cos(pitch)*sin(roll)*euler_yaw_rate_setpoint;

== matlab function FixedWing_Dynamic_Model_SIL_simulink/Controllers/Attitude Controller/MATLAB Function4 ==
  data: roll input; yaw_body_rate_setpoint_raw output; pitch input; euler_pitch_rate_setpoint input; euler_rate_setpoint_yaw input
function yaw_body_rate_setpoint_raw    = yaw_crtl(roll,pitch,euler_pitch_rate_setpoint,euler_rate_setpoint_yaw)

yaw_body_rate_setpoint_raw = -sin(roll)*euler_pitch_rate_setpoint+cos(roll)*cos(pitch)*euler_rate_setpoint_yaw;

== matlab function FixedWing_Dynamic_Model_SIL_simulink/Controllers/MATLAB Function1 ==
  data: tas_error_percentage input; ratio_undersped output; equivalent_airspeed_trim input; tas_min input; tas input
function ratio_undersped = ratio_underspeed(tas_error_percentage,equivalent_airspeed_trim,tas_min,tas)

tas_error_bound = tas_error_percentage*equivalent_airspeed_trim;
tas_undersped_soft_bound = tas_error_bound*equivalent_airspeed_trim;

tas_fully_undersped = max(tas_min-tas_error_bound-tas_undersped_soft_bound,0);
tas_starting_to_undersped = max(tas_min-tas_error_bound,tas_fully_undersped);

ratio_undersped = 1-((norm(tas)-tas_fully_undersped)/max(tas_starting_to_undersped-tas_fully_undersped,10^-6));

== matlab function FixedWing_Dynamic_Model_SIL_simulink/Controllers/Attitude Controller/MATLAB Function5 ==
  data: roll input; euler_rate_setpoint_yaw output; euler_rate_setpoint_pitch output; roll_setpoint input; pitch input; airspeed input; pitch_setpoint input; tc input
function [euler_rate_setpoint_yaw,euler_rate_setpoint_pitch] = euler_rate(roll,roll_setpoint,pitch,airspeed,pitch_setpoint,tc)
g = 9.81;
contrained_roll = min(max(roll,-abs(roll_setpoint)),abs(roll_setpoint));
euler_rate_setpoint_yaw = tan(contrained_roll)*cos(pitch)*g/airspeed; % turn coordination

pitch_error = pitch_setpoint-pitch;
euler_rate_setpoint_pitch = pitch_error/tc;

== matlab function FixedWing_Dynamic_Model_SIL_simulink/Controllers/Total Energy control system/Total energy control loop/MATLAB Function4 ==
  data: throttle_max input; throttle_min input; throttle_integ_input input; throttle_integ_state output
function throttle_integ_state = T_integ(throttle_max,throttle_min, throttle_integ_input)

if throttle_integ_input >= throttle_max
    throttle_integ_input = min(0,throttle_integ_input);
elseif throttle_integ_input<= throttle_min
    throttle_integ_input = max(0,throttle_integ_input);
end
    throttle_integ_state = throttle_integ_input;

== matlab function FixedWing_Dynamic_Model_SIL_simulink/Controllers/Total Energy control system/Total energy balance control loop/MATLAB Function4 ==
  data: vert_accel_limit input; pitch_increment output; V_TAS input
function pitch_increment = pitch_incre(vert_accel_limit,V_TAS)

pitch_increment = vert_accel_limit / max(V_TAS,10^-6);

== matlab function FixedWing_Dynamic_Model_SIL_simulink/Controllers/Total Energy control system/Total energy balance control loop/MATLAB Function5 ==
  data: pitch_setpoint input; pitch_increment input; pitch_setpoint output
function pitch_setpoint = pitch_incre_lim(pitch_setpoint,pitch_increment)
pitch_setpoint = min(max(pitch_setpoint,pitch_setpoint-pitch_increment),pitch_setpoint+pitch_increment);

== matlab function FixedWing_Dynamic_Model_SIL_simulink/Controllers/MATLAB Function4 ==
  data: ratio_undersped input; weight_spe output; pitch_speed_weight input; weight_ske output
function [weight_spe,weight_ske] = weight(ratio_undersped,pitch_speed_weight)

pitch_speed_weight = min(max(pitch_speed_weight,0),2);

if ratio_undersped>10^-6
    pitch_speed_weight = 2*ratio_undersped+(1-ratio_undersped)*pitch_speed_weight;
end

weight_spe = min(max(2-pitch_speed_weight,0),1);
weight_ske = min(max(pitch_speed_weight,0),1);

== matlab function FixedWing_Dynamic_Model_SIL_simulink/Controllers/Total Energy control system/Total energy control loop/MATLAB Function2 ==
  data: ste_rate input; ste_rate_max input; T_FF output; ste_rate_min input; throttle_max input; throttle_min input; throttle_trim input
function T_FF  = T_predicted(ste_rate,ste_rate_max, ste_rate_min, throttle_max, throttle_min, throttle_trim)
throttle_above_trim_per_ste_rate = (throttle_max - throttle_trim)/ste_rate_max;
throttle_below_trim_per_ste_rate = (throttle_trim - throttle_min)/ste_rate_min;

if ste_rate >= 10^-6
    T_FF = throttle_trim + ste_rate*throttle_above_trim_per_ste_rate;
else
    T_FF = throttle_trim - ste_rate*throttle_below_trim_per_ste_rate;
end

== matlab function FixedWing_Dynamic_Model_SIL_simulink/Controllers/Total Energy control system/Total energy balance control loop/MATLAB Function2 ==
  data: SEB_rate_correction input; pitch_setpoint_1 output; V_TAS input
function pitch_setpoint_1  = seb_to_pitch(SEB_rate_correction,V_TAS)

g = 9.81;
airspeed_for_seb_rate = 15;

if V_TAS > 10^-6

airspeed_for_seb_rate = V_TAS;
end 

climb_angle_to_SEB_rate = airspeed_for_seb_rate*g;

pitch_setpoint_1 = SEB_rate_correction/climb_angle_to_SEB_rate;

== matlab function FixedWing_Dynamic_Model_SIL_simulink/Controllers/Seguimiento waypoints/MATLAB Function4 ==
  data: Vcruise input; velocidad output; current_wp input; poswp input; nwap input
function velocidad  = vel(Vcruise, current_wp,poswp,nwap)

velocidad = Vcruise(1);
for i = 1:nwap
    if current_wp(1) == poswp(i,1)
        velocidad = Vcruise(i);
    end
end

== matlab function FixedWing_Dynamic_Model_SIL_simulink/Controllers/MATLAB Function ==
  data: vxyz input; course output; gndspeed output
function [course, gndspeed] = cour_gnds(vxyz)

vx = vxyz(1);
vy = vxyz(2);

course = atan2(vy,vx);
gndspeed = norm([vx,vy]);

== matlab function FixedWing_Dynamic_Model_SIL_simulink/Controllers/Total Energy control system/Total energy balance control loop/MATLAB Function3 ==
  data: pitch_max input; pitch_integ_state output; pitch_min input; pitch_integ_input input
function pitch_integ_state = p_integ(pitch_max,pitch_min,pitch_integ_input)
if pitch_integ_input >= pitch_max
    pitch_integ_input = min(pitch_integ_input,0);
elseif pitch_integ_input <= pitch_min
    pitch_integ_input = max(pitch_integ_input,0);
end
pitch_integ_state = pitch_integ_input;

== matlab function FixedWing_Dynamic_Model_SIL_simulink/Controllers/Seguimiento waypoints/MATLAB Function2 ==
  data: toWP input; wps output; fromWP input; alt output
function [wps, alt]= waypoints_alt(toWP, fromWP)
    wps = zeros(2,3); 
    wps = [fromWP'; toWP'];
    alt = -toWP(3);
end

== matlab function FixedWing_Dynamic_Model_SIL_simulink/Controllers/MATLAB Function2 ==
  data: max_climb_rate input; ste_rate_to_throttle output; min_sink_rate input; ste_rate_max output; ste_rate_min output
function [ste_rate_to_throttle,ste_rate_max,ste_rate_min]  = ste(max_climb_rate,min_sink_rate)
 g = 9.81;
ste_rate_max = max(max_climb_rate,10^-6)*g;
ste_rate_min = -max(min_sink_rate,10^-6)*g;

ste_rate_to_throttle = 1/(ste_rate_max-ste_rate_min);

== matlab function FixedWing_Dynamic_Model_SIL_simulink/Controllers/MATLAB Function3 ==
  data: ste_rate_max input; airspeed_rate_output output; ste_rate_min input; V_TAS input; airspeed_rate input
function airspeed_rate_output = V_rate(ste_rate_max,ste_rate_min,V_TAS,airspeed_rate)
max_tas_rate_sp = 0.5*ste_rate_max/max(V_TAS,10^-6);
min_tas_rate_sp = 0.5*ste_rate_min/max(V_TAS,10^-6);

airspeed_rate_output = min(max(airspeed_rate,min_tas_rate_sp),max_tas_rate_sp);
